simulink model "ctc_ut"  (Simulink 8.1)
settings: Solver=FixedStepDiscrete  StartTime=0.0  StopTime=10  FixedStep=0.005  RelTol=1e-3
PostLoadFcn:
  | , if any(exist('dsrtsu_mdlpostloadfcn', 'file') == [2, 3, 6]), try dsrtsu_mdlpostloadfcn('Execute', bdroot); catch fprintf('Error in PostLoadFcn (dsrtsu_mdlpostloadfcn) for model "%s":\n %s\n', bdroot, lasterr); end, end,
libraries: siltestlib x21, ctc x1
settings Model: DSRTSU_INTERNAL_RTI_VER=450  DSRTSU_INTERNAL_RTI_TYPE=rti1401  RTICANMMDATA=struct('GeneralSetupData',struct('modelroot','D:\ELN150201_TAIWAN\trunk\AdasDragon\software\sw_development\arch\app\acc','generalsettings',struct('filesettings',struct('destfolder',struct('Name','RTICANMM_FILES','Check',1),'buildfolder',struct('Name','.','Check',1),'AbsDestfolder',struct('Name','D:\ELN150201_TAIWAN\trunk\AdasDragon\software\sw_development\arch\app\acc\RTICANMM_FILES'),'AbsBuildfolder',struct('Name','D:\ELN150201_TAIWAN\trunk\AdasDragon\software\sw_development\arch\app\acc'))),'options',struct('addpaths',1,'rmpaths',1,'addtrcexclusion',logical(1),'cannavigator',struct('checkmonitoring',0),'show_usrtrc',0,'use_usrtrc',0),'advanced',struct('options',[1 1 1 1 1 1 1 1 1 1 1 1 1 1 1 1 1 1 1 1 1 1 1 1 1 1 1 1 1 1 1 1 1 1 1 1 1 1 1 1 1 1 1 1 1 1 1 1 1 1 1 1 1 1 1 1 1 1 1 1 1 1 1 1 1 1 1 1 1 1 1 1 1 1 1 1 1 1 1 1 1 1 1 1 1 1 1 1 1 1 1 1 1 1 1 1 1 1 1 1]),'MPSetup',{{}},'modelname','ctc_ut','block','ctc_ut'))  DSRTSU_INTERNAL_RTIFPGA=40  Creator=AT015411  LastModifiedBy=AT015555  BufferReuse=off
settings DataIOCC: SignalLoggingSaveFormat=Dataset
settings OptimizationCC: BlockReduction=off  OptimizeBlockIOStorage=off  BufferReuse=off  ExpressionFolding=off  ExpressionDepthLimit=128  LocalBlockOutputs=off
settings DebuggingCC: FcnCallInpInsideContextMsg=EnableAllAsError
settings HardwareCC: ProdIntDivRoundTo=Zero  ProdEndianess=BigEndian  ProdHWDeviceType=Generic->Custom  TargetIntDivRoundTo=Zero  TargetEndianess=BigEndian  TargetHWDeviceType=Generic->Custom
settings RTWCC: SystemTargetFile=rti1005.tlc  MakeCommand=make_rti  TemplateMakefile=rti1005.tmf  Description=dSPACE DS1005 Hardware Platform  ProcessScript=rti1005_make_rtw_hook
settings STFCustomTargetCC: CodeReplacementLibrary=ANSI_C  ParMdlRefBuildCompliant=on  GeneratePreprocessorConditionals=Disable all  MatFileLogging=on  SystemTargetFile=rti1005.tlc
settings GRTTargetCC: CompOptLevelCompliant=off  ConcurrentExecutionCompliant=off  ExtModeMexFile=noextcomm
settings CustomProperty: DataType=RTWOptions_EnumType_C__Program Files (x86)_dSPACE RCPHIL 2014-B_MATLAB_RTI_RTI1401_TLC_rti1005_1InitialSimState  Value=RUN
settings EnumStrPairs: String=RUN

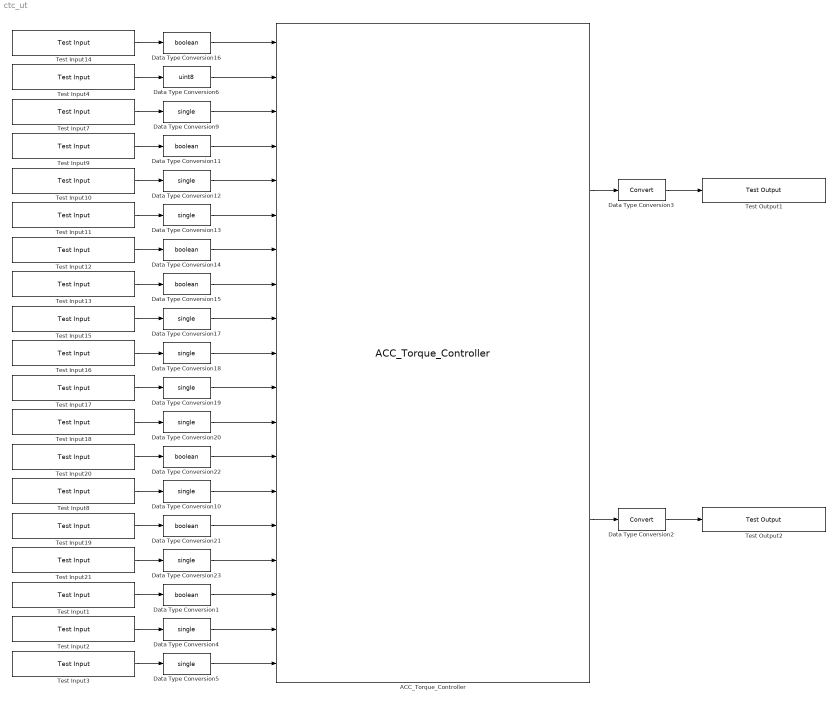
== system ctc_ut ==
  ACC_Torque_Controller : ctc/ACC_Torque_Controller
  Data Type Conversion{1,11,14..16,21..22} (7 alike) : DataTypeConversion  OutDataTypeStr=boolean
  Data Type Conversion{4..5,9..10,12..13,17..20,23} (11 alike) : DataTypeConversion  OutDataTypeStr=single
  Data Type Conversion2 : DataTypeConversion
  Data Type Conversion3 : DataTypeConversion
  Data Type Conversion6 : DataTypeConversion  OutDataTypeStr=uint8
  Test Input1 : siltestlib/Test Input  varname=VACC_ACCDistControlSel_flg  sampletime=0.005
  Test Input10 : siltestlib/Test Input  varname=VJUD_VehSpd_kph  sampletime=0.005
  Test Input11 : siltestlib/Test Input  varname=VDINR_CurDriverTqReq_Nm  sampletime=0.005
  Test Input12 : siltestlib/Test Input  varname=VIFO_ACCSetSpdDec_flg  sampletime=0.005
  Test Input13 : siltestlib/Test Input  varname=VIFO_ACCResSpdInc_flg  sampletime=0.005
  Test Input14 : siltestlib/Test Input  varname=VIFO_DriverTurnSignalOn_flg  sampletime=0.005
  Test Input15 : siltestlib/Test Input  varname=VDINR_EngTqMax_Nm  sampletime=0.005
  Test Input16 : siltestlib/Test Input  varname=VDINR_EngTqMin_Nm  sampletime=0.005
  Test Input17 : siltestlib/Test Input  varname=VDINR_LongAccel_G  sampletime=0.005
  Test Input18 : siltestlib/Test Input  varname=VDINR_LatAccel_G  sampletime=0.005
  Test Input19 : siltestlib/Test Input  varname=VACC_TorqueReleaseReq_flg  sampletime=0.005
  Test Input2 : siltestlib/Test Input  varname=VACC_ACCDecelReqPrev_mps2  sampletime=0.005
  Test Input20 : siltestlib/Test Input  varname=VACC_ACCTargetVehAssigned_flg  sampletime=0.005
  Test Input21 : siltestlib/Test Input  varname=VACC_ACCRefSpd_mps  sampletime=0.005
  Test Input3 : siltestlib/Test Input  varname=VACC_DesiredDistance_m  sampletime=0.005
  Test Input4 : siltestlib/Test Input  varname=VACC_ACCSystemState_enum  sampletime=0.005
  Test Input7 : siltestlib/Test Input  varname=VDINR_EngTqIndicated_Nm  sampletime=0.005
  Test Input8 : siltestlib/Test Input  varname=VACC_VehSpd_mps  sampletime=0.005
  Test Input9 : siltestlib/Test Input  varname=VACC_ACCOverride_flg  sampletime=0.005
  Test Output1 : siltestlib/Test Output  varname=VACC_ACCTorqueReq_Nm  sampletime=-1
  Test Output2 : siltestlib/Test Output  varname=VACC_ACCRawTorqueReq_Nm  sampletime=-1
  wires:
  Data Type Conversion2/1 -> Test Output2/1
  ACC_Torque_Controller/2 -> Data Type Conversion2/1
  Data Type Conversion3/1 -> Test Output1/1
  ACC_Torque_Controller/1 -> Data Type Conversion3/1
  Test Input7/1 -> Data Type Conversion9/1
  Test Input8/1 -> Data Type Conversion10/1
  Test Input9/1 -> Data Type Conversion11/1
  Test Input10/1 -> Data Type Conversion12/1
  Test Input11/1 -> Data Type Conversion13/1
  Test Input12/1 -> Data Type Conversion14/1
  Test Input13/1 -> Data Type Conversion15/1
  Test Input14/1 -> Data Type Conversion16/1
  Test Input15/1 -> Data Type Conversion17/1
  Data Type Conversion17/1 -> ACC_Torque_Controller/9
  Test Input16/1 -> Data Type Conversion18/1
  Data Type Conversion18/1 -> ACC_Torque_Controller/10
  Test Input17/1 -> Data Type Conversion19/1
  Data Type Conversion19/1 -> ACC_Torque_Controller/11
  Test Input18/1 -> Data Type Conversion20/1
  Data Type Conversion20/1 -> ACC_Torque_Controller/12
  Test Input19/1 -> Data Type Conversion21/1
  Test Input20/1 -> Data Type Conversion22/1
  Test Input21/1 -> Data Type Conversion23/1
  Data Type Conversion21/1 -> ACC_Torque_Controller/15
  Data Type Conversion22/1 -> ACC_Torque_Controller/13
  Data Type Conversion23/1 -> ACC_Torque_Controller/16
  Data Type Conversion12/1 -> ACC_Torque_Controller/5
  Data Type Conversion13/1 -> ACC_Torque_Controller/6
  Data Type Conversion14/1 -> ACC_Torque_Controller/7
  Data Type Conversion15/1 -> ACC_Torque_Controller/8
  Data Type Conversion10/1 -> ACC_Torque_Controller/14
  Data Type Conversion11/1 -> ACC_Torque_Controller/4
  Data Type Conversion9/1 -> ACC_Torque_Controller/3
  Test Input1/1 -> Data Type Conversion1/1
  Data Type Conversion1/1 -> ACC_Torque_Controller/17
  Test Input2/1 -> Data Type Conversion4/1
  Test Input3/1 -> Data Type Conversion5/1
  Data Type Conversion4/1 -> ACC_Torque_Controller/18
  Data Type Conversion5/1 -> ACC_Torque_Controller/19
  Test Input4/1 -> Data Type Conversion6/1
  Data Type Conversion16/1 -> ACC_Torque_Controller/1
  Data Type Conversion6/1 -> ACC_Torque_Controller/2
